simulink model "wash"  (R2024b)
settings: Solver=VariableStepAuto  StartTime=0.0  StopTime=10.0  RelTol=1e-3
settings Model: Creator=Pramod C  LastModifiedBy=Pramod C

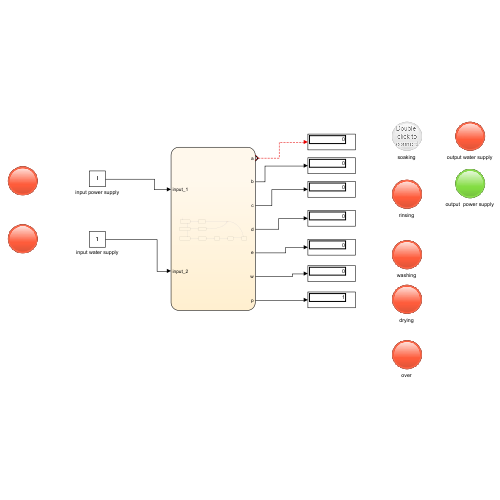
[thumbnail: Simulink's stored preview of the top-level diagram]
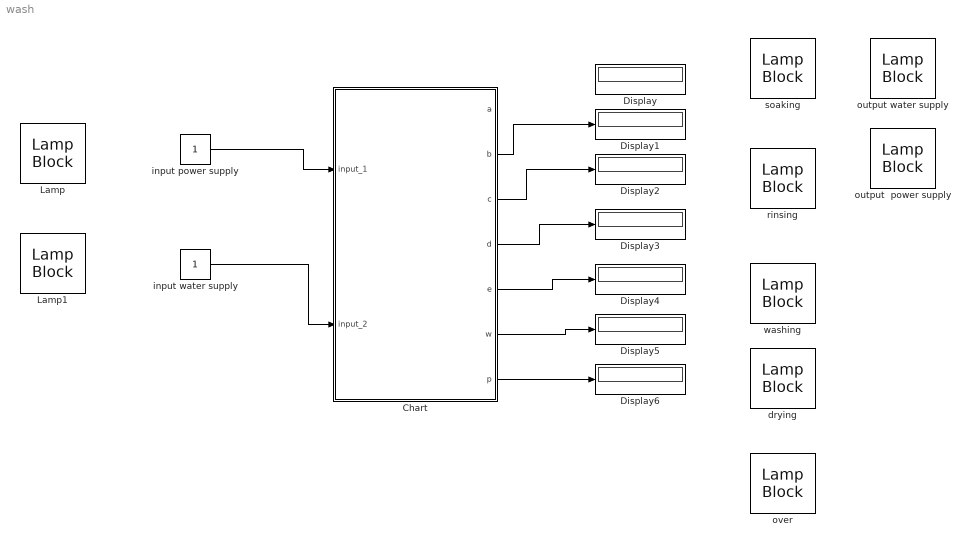
== system wash ==
  Chart : Stateflow chart  TreatAsAtomicUnit=on
  Display{,1..6} (7 alike) : Display
  Lamp : LampBlock  LabelPosition=Hide
  Lamp1 : LampBlock  LabelPosition=Hide
  drying : LampBlock  LabelPosition=Hide
  input power supply : Constant
  input water supply : Constant
  output  power supply : LampBlock  LabelPosition=Hide
  output water supply : LampBlock  LabelPosition=Hide
  over : LampBlock  LabelPosition=Hide
  rinsing : LampBlock  LabelPosition=Hide
  soaking : LampBlock  LabelPosition=Hide
  washing : LampBlock  LabelPosition=Hide
  wires:
  input power supply/1 -> Chart/1(input_1)
  input water supply/1 -> Chart/2(input_2)
  ? -> Display/1
  Chart/2(b) -> Display1/1
  Chart/3(c) -> Display2/1
  Chart/4(d) -> Display3/1
  Chart/5(e) -> Display4/1
  Chart/6(w) -> Display5/1
  Chart/7(p) -> Display6/1

== stateflow chart wash/Chart ==
  state Power_supply_on
    entry: p=1
  state Power_supply_off
  state Water_supply_on
    entry: w=1
  state Water_supply_off
  state Filling
    entry: a=1
    exit:a=0
  state Washing
    entry:b=1
    exit: b=0
  state Rinsing
    entry: c=1
    exit: c=0;
    exit: w=0;
  state Spining
    entry: d=1
    exit: d=0
  state Done
    entry: e=1
    exit: p=0
  (default) -> Power_supply_on
  Power_supply_on -> Power_supply_off [order 1] : [input_1==0]
  Power_supply_off -> (junction 21)
  Done -> (junction 21)
  Water_supply_off -> (junction 21)
  Power_supply_on -> Water_supply_on [order 2] : [input_1==0]
  Water_supply_on -> Water_supply_off [order 1] : [input_2==0]
  Water_supply_on -> Filling [order 2] : [input_2==0]
  Spining -> Done : after(50,sec)
  Filling -> Washing : after(200,sec)
  Washing -> Rinsing : after (100,sec)
  Rinsing -> Spining : after(20,sec)
  data: a output; input_1 input; input_2 input; b output double; c output double; d output double; e output double; w output double; p output double
